simulink model "simple_example"  (R2021a)
settings: Solver=VariableStepAuto  StartTime=0.0  StopTime=10  MaxStep=0.01  RelTol=1e-16
libraries: adrc_toolbox_library x1
settings Model: Creator=krzys  LastModifiedBy=krzys

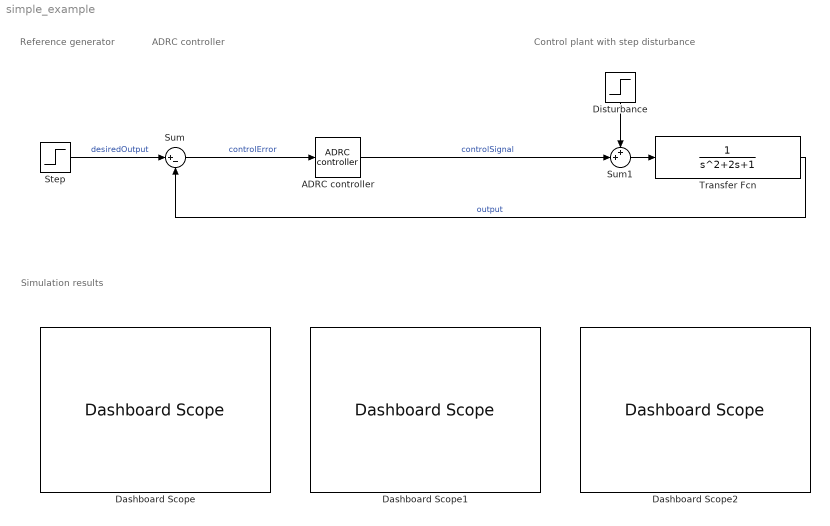
== system simple_example ==
  note: Simulation results
  note: Reference
      | generator
  note: ADRC controller
  note: Control plant with step disturbance
  ADRC controller : adrc_toolbox_library/ADRC controller  dynamicsOrder=2  inputGainParameter=0.85  controllerBandwidth=5  observerBandwidth=25
      settings: SourceProductName=ADRC toolbox
  Dashboard Scope : DashboardScope
  Dashboard Scope1 : DashboardScope
  Dashboard Scope2 : DashboardScope
  Disturbance : Step  Time=5  SampleTime=0
  Step : Step  SampleTime=0
  Sum : Sum  Inputs=|+-
  Sum1 : Sum  Inputs=++|
  Transfer Fcn : TransferFcn
  wires:
  Step/1 -> Sum/1  "desiredOutput"
  Sum/1 -> ADRC controller/1  "controlError"
  Transfer Fcn/1 -> Sum/2  "output"
  Sum1/1 -> Transfer Fcn/1
  Disturbance/1 -> Sum1/1
  ADRC controller/1 -> Sum1/2  "controlSignal"
